simulink model "fluidMechanicsSim"  (R2025b)
settings: Solver=VariableStepAuto  StartTime=0.0  StopTime=10  RelTol=1e-3
undefined symbols (not defined in the file or in its folder): constantsSTADPOLE
settings Model: Creator=Eric  LastModifiedBy=alex2

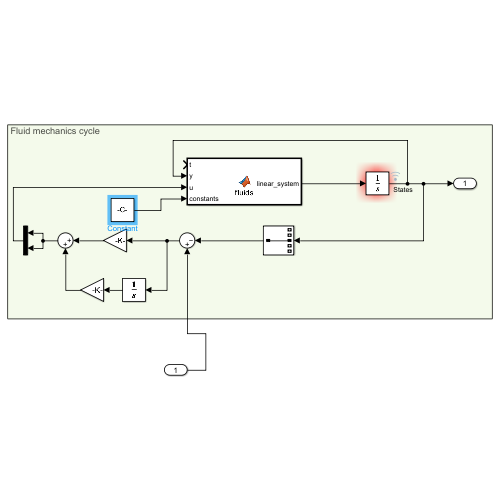
[thumbnail: Simulink's stored preview of the top-level diagram]
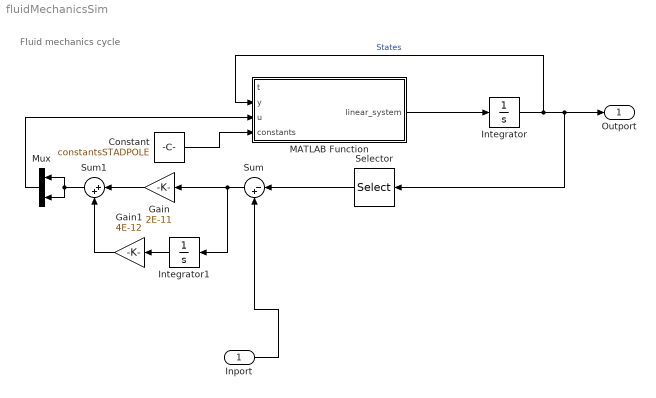
== system fluidMechanicsSim ==
  note: Fluid mechanics cycle
  Inport : Inport
  Constant : Constant  Value=constantsSTADPOLE
  Gain : Gain  Gain=2E-11
  Gain1 : Gain  Gain=4E-12
  Integrator : Integrator  InitialCondition=constantsSTADPOLE.init_cond
  Integrator1 : Integrator
  MATLAB Function : MATLAB Function  TreatAsAtomicUnit=on
  Mux : Mux  Inputs=2
  Selector : Selector  InputPortWidth=5  IndexOptions=Index vector (dialog)  Indices=3  OutputSizes=1
  Sum : Sum  Inputs=|-+
  Sum1 : Sum  Inputs=|++
  Outport : Outport
  wires:
  Integrator/1 -> MATLAB Function/2(y), Outport/1, Selector/1  "States"
  MATLAB Function/1(linear_system) -> Integrator/1
  Selector/1 -> Sum/1
  Sum/1 -> Integrator1/1, Gain/1
  Mux/1 -> MATLAB Function/3(u)
  Integrator1/1 -> Gain1/1
  Gain1/1 -> Sum1/2
  Gain/1 -> Sum1/1
  Sum1/1 -> Mux/1, Mux/2
  Inport/1 -> Sum/2
  Constant/1 -> MATLAB Function/4(constants)

== matlab function fluidMechanicsSim/MATLAB Function ==
  data: t input; linear_system output; y input; u input; constants input
function linear_system = fluids(t,y,u, constants)
    linear_system = fluidMechanics(t,y,u,constants);
end
